simulink model "detectorSimulink"  (R2019b)
settings: Solver=VariableStepAuto  StartTime=0.0  StopTime=10.0  RelTol=1e-3
undefined symbols (not defined in the file or in its folder): none
libraries: visiontextngfix x1, dspvision x1, imaqlib x1
settings Model: Creator=mustafa  LastModifiedBy=mustafa

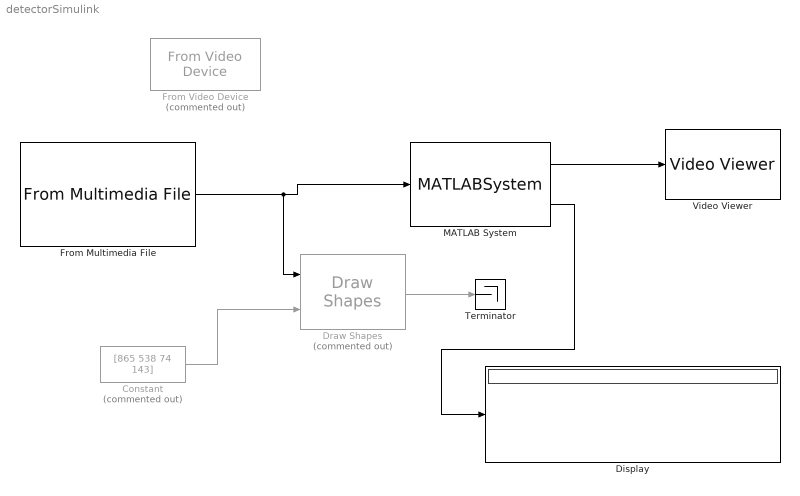
== system detectorSimulink ==
  Constant : Constant  Commented=on  Value=[865 538 74 143]
  Display : Display
  Draw Shapes : visiontextngfix/Draw Shapes  Commented=on  shape=Rectangles  fill=off  lineWidth=1  fillClrSource=Specify via dialog  display=Black  intensity=200  color=[200 255 100]  opacity=0.6  viewport=Entire image  antialiasing=off  inType=Obsolete  imagePorts=One multidimensional signal  roundingMode=Floor  overflowMode=off  memoryMode=Specify word length  memoryWordLength=16  prodOutputMode=Binary point scaling  prodOutputWordLength=32  prodOutputFracLength=14  prodOutputSlope=2^-14  accumSlope=2^-14  memoryFracLength=15
      settings: SourceProductName=Computer Vision Toolbox
  From Multimedia File : dspvision/From Multimedia File  inputFilename=/Users/mustafa/Documents/MATLAB/222.avi  readRange=[1 Inf]  loop=on  numPlays=1  outputStreams=Video only  videoDataType=uint8  audioDataType=int16  inheritSampleTime=on  userDefinedSampleTime=1/30  noAudioOutput=off  isIntensityVideo=off  fourcc=RGB  colorVideoFormat=One multidimensional signal  outputEOF=off  dataOrg=Column-major  audioFrameSize=1024  computeAudioFrameSize=off  outSamplingMode=Sample based
      settings: SourceProductName=DSP System Toolbox  SourceProductBaseCode=DS
  From Video Device : imaqlib/From Video Device  Commented=on  DeviceMenu=(none)  Device=(none)  ObjConstructor=(none)  VideoFormatMenu=(none)  VideoFormat=(none)  VideoSource=none  ROIPosition=(none)  EnableHWTrigger=off  TriggerConfiguration=none/none  SampleTime=1/30  OutputPortsMode=One multidimensional signal  DataType=single  CanDoHWTrigger=no  ReturnedColorSpace=rgb  BlockHandle=50.0012  ROIWidth=100  ROIHeight=100  ROIColumn=0  ROIRow=0  EngXMLPath=/Applications/MATLAB_R2019b.app/toolbox/imaq/imaq/private  DevXMLPath=DEVPATH  EngLibPath=/Applications/MATLAB_R2019b.app/toolbox/imaq/imaqblks/imaqmex/maci64  ColorSpace=rgb  BayerSensorAlignment=grbg  ImaqMode=off
      settings: SourceProductName=Image Acquisition Toolbox
  MATLAB System : MATLABSystem  System=detectorSim  numberOfVehicles=[2]  SimulateUsing=Interpreted execution
      mask Type: detectorSim
      mask Display:
      | disp('detectorSim');
      | port_label('input',1,'I');
      | port_label('output',1,'y');
      | port_label('output',2,'bboxes');
  Terminator : Terminator
  Video Viewer : VideoViewer  FigPos=[291 1011 1440 711]
  wires:
  From Multimedia File/1 -> Draw Shapes/1, MATLAB System/1
  Constant/1 -> Draw Shapes/2
  MATLAB System/1 -> Video Viewer/1
  Draw Shapes/1 -> Terminator/1
  MATLAB System/2 -> Display/1
